simulink library "Lib_Solve_NormErr_TMATS"  (R2015a)
settings: Solver=ode45  StartTime=0.0  StopTime=10.0  RelTol=1e-3
Description:
  | Thomas Modules
settings Model: Creator=jwchapm2  LastModifiedBy=jwchapm2
settings OptimizationCC: ExpressionDepthLimit=2147483647
settings DebuggingCC: UnderspecifiedInitializationDetection=Classic  MergeDetectMultiDrivingBlocksExec=none  SolverPrmCheckMsg=warning  StateNameClashWarn=warning

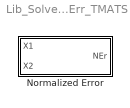
== system Lib_Solve_NormErr_TMATS ==
  Normalized Error : Subsystem  mask(T-MATS: Normalized Error Library Block){}
      mask help:
      | This block offers an easy way to add a normalized error to be used with the solvers.
      |
      | (X1 - X2)/X1 = NEr
      mask Help: web(which('Solver_TMATS_NEr.html'),'-helpbrowser')

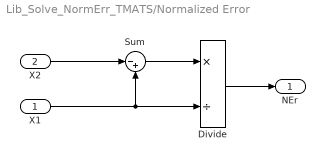
== system Lib_Solve_NormErr_TMATS/Normalized Error ==
  X1 : Inport
  X2 : Inport  Port=2
  Divide : Product  Inputs=*/
  Sum : Sum  Inputs=|-+
  NEr : Outport
  wires:
  X2/1 -> Sum/1
  X1/1 -> Divide/2, Sum/2
  Divide/1 -> NEr/1
  Sum/1 -> Divide/1
